simulink library "dspadpt2"  (Simulink 3.00)
libraries: simulink3 x5, dspbdsp2 x5, dspmtrx2 x5, dspbuff2 x3, dspvect2 x1
settings Model: Creator=don  LastModifiedBy=sconahan

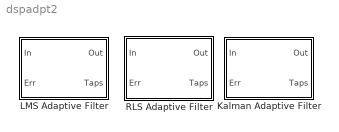
== system dspadpt2 ==
  Kalman Adaptive Filter : Subsystem  mask(Kalman Adaptive Filter){Ntaps=5, Jmin=0.3, q=0.1, ic0=0, K0=0.5, Adapt=off}
      mask prompts: Ntaps "FIR filter length:"; Jmin "Measurement noise variance:"; q "Process noise variance:"; ic0 "Initial value of filter taps:"; K0 "Initial error correlation matrix:"; Adapt "Adapt input"
      mask help: One-step Kalman predictor algorithm for adaptive FIR filtering of input signal. If Adapt input checkbox is enabled, and the Adapt input port is zero, the algorithm stops adapting the filter coefficients.
      mask init:
      | if prod(size(ic0))==1, ic = ic0(ones(Ntaps,1)); else ic = ic0; end
      | if prod(size(K0))==1, K = K0.*eye(Ntaps);
      | elseif any(size(K0)==1), K = diag(K0);
      | else K=K0; end
      | dspblkadpt('init');
      mask Help: web(dspbhelp);
      mask Display: disp('Kalman')
  LMS Adaptive Filter : Subsystem  mask(LMS Adaptive Filter){n=32, mu=.65, ic=0.0, normalized=on, Adapt=off}
      mask prompts: n "FIR filter length:"; mu "Step-size, mu:"; ic "Initial value of filter taps:"; normalized "Use normalization"; Adapt "Adapt input"
      mask help: Least mean-square (LMS) algorithm for adaptive FIR filtering of input signal. Energy normalization may optionally be disabled. If Adapt input checkbox is enabled, and the Adapt input port is zero, the algorithm stops adapting the filter coefficients.
      mask init:
      | if normalized, s='nLMS'; else s='LMS'; end
      | dspblkadpt('init');
      mask Help: web(dspbhelp);
      mask Display: disp(s);
  RLS Adaptive Filter : Subsystem  mask(RLS Adaptive Filter){Ntaps=32, Lambda=1.0, ic=0.0, phi0=0.1, Adapt=off}
      mask prompts: Ntaps "FIR filter length:"; Lambda "Memory weighting factor (0 to 1):"; ic "Initial value of filter taps:"; phi0 "Initial input variance estimate:"; Adapt "Adapt input"
      mask help: Exponentially weighted recursive least-squares (RLS) algorithm for adaptive FIR filtering of input signal. If Adapt input checkbox is enabled, and the Adapt input port is zero, the algorithm stops adapting the filter coefficients.
      mask init:
      | dspblkadpt('init');
      mask Help: web(dspbhelp);
      mask Display: disp('RLS')

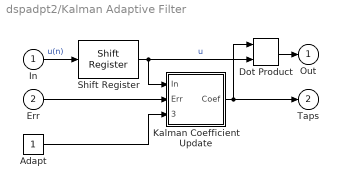
== system dspadpt2/Kalman Adaptive Filter ==
  In : Inport  Port=1  PortWidth=-1  SampleTime=-1  DataType=auto
      settings: SignalType=auto
  Err : Inport  Port=2  PortWidth=-1  SampleTime=-1  DataType=auto
      settings: SignalType=auto
  Adapt : Constant  Value=1
  Dot Product : simulink3/Math/Dot Product
  Kalman Coefficient Update : Subsystem
  Shift Register : dspbuff2/Shift Register  siz=Ntaps  ic=0
  Out : Outport  Port=1  InitialOutput=0
  Taps : Outport  Port=2  InitialOutput=0
  wires:
  In/1 -> Shift Register/1  "u(n)"
  Dot Product/1 -> Out/1
  Err/1 -> Kalman Coefficient Update/2(Err)
  Adapt/1 -> Kalman Coefficient Update/3(Adapt)
  Shift Register/1 -> Kalman Coefficient Update/1(In), Dot Product/2  "u"
  Kalman Coefficient Update/1(Coef) -> Taps/1, Dot Product/1

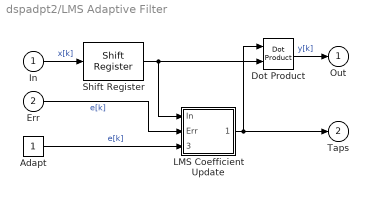
== system dspadpt2/LMS Adaptive Filter ==
  In : Inport  Port=1  PortWidth=-1  SampleTime=-1  DataType=auto
      settings: SignalType=auto
  Err : Inport  Port=2  PortWidth=-1  SampleTime=-1  DataType=auto
      settings: SignalType=auto
  Adapt : Constant  Value=1
  Dot Product : simulink3/Math/Dot Product
  LMS Coefficient Update : Subsystem
  Shift Register : dspbuff2/Shift Register  siz=n  ic=0
  Out : Outport  Port=1  InitialOutput=0
  Taps : Outport  Port=2  InitialOutput=0
  wires:
  Dot Product/1 -> Out/1  "y[k]"
  In/1 -> Shift Register/1  "x[k]"
  Err/1 -> LMS Coefficient Update/2(Err)  "e[k]"
  Adapt/1 -> LMS Coefficient Update/3(Adapt)  "e[k]"
  LMS Coefficient Update/1(Coef) -> Taps/1, Dot Product/1
  Shift Register/1 -> LMS Coefficient Update/1(In), Dot Product/2

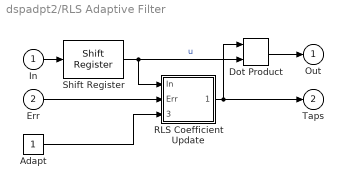
== system dspadpt2/RLS Adaptive Filter ==
  In : Inport  Port=1  PortWidth=-1  SampleTime=-1  DataType=auto
      settings: SignalType=auto
  Err : Inport  Port=2  PortWidth=-1  SampleTime=-1  DataType=auto
      settings: SignalType=auto
  Adapt : Constant  Value=1
  Dot Product : simulink3/Math/Dot Product
  RLS Coefficient Update : Subsystem
  Shift Register : dspbuff2/Shift Register  siz=Ntaps  ic=0
  Out : Outport  Port=1  InitialOutput=0
  Taps : Outport  Port=2  InitialOutput=0
  wires:
  In/1 -> Shift Register/1
  Dot Product/1 -> Out/1
  Err/1 -> RLS Coefficient Update/2(Err)
  Adapt/1 -> RLS Coefficient Update/3(Adapt)
  RLS Coefficient Update/1(Coef) -> Taps/1, Dot Product/1
  Shift Register/1 -> RLS Coefficient Update/1(In), Dot Product/2  "u"

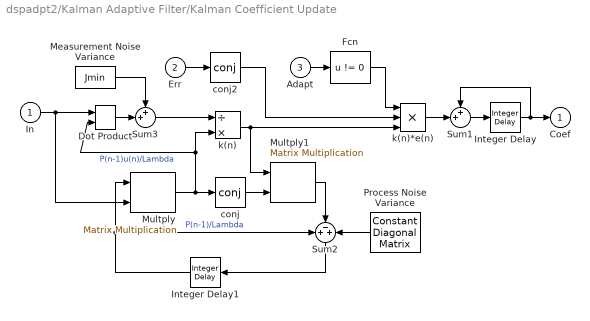
== system dspadpt2/Kalman Adaptive Filter/Kalman Coefficient Update ==
  In : Inport  Port=1  PortWidth=-1  SampleTime=-1  DataType=auto
      settings: SignalType=auto
  Err : Inport  Port=2  PortWidth=-1  SampleTime=-1  DataType=auto
      settings: SignalType=auto
  Adapt : Inport  Port=3  PortWidth=-1  SampleTime=-1  DataType=auto
      settings: SignalType=auto
  Dot Product : simulink3/Math/Dot Product
  Fcn : Fcn  Expr=u != 0
  Integer Delay : dspbdsp2/Integer Delay  delay=1  ic=ic  frame=off  df=on  numChans=1
  Integer Delay1 : dspbdsp2/Integer Delay  Orientation=left  delay=1  ic=K  frame=off  df=on  numChans=1
  Measurement Noise Variance : Constant  Value=Jmin
  Multply : dspmtrx2/Matrix Multiplication  Asize=[Ntaps Ntaps]  Bcols=1
  Multply1 : dspmtrx2/Matrix Multiplication  Asize=[Ntaps 1]  Bcols=Ntaps
  Process Noise Variance : dspmtrx2/Constant Diagonal Matrix  Orientation=left  n=Ntaps  q=q
  Sum1 : Sum  Inputs=++|  SaturateOnIntegerOverflow=on
  Sum2 : Sum  Orientation=down  Inputs=+-+  SaturateOnIntegerOverflow=on
  Sum3 : Sum  Inputs=++|  SaturateOnIntegerOverflow=on
  conj : Math  Operator=conj  OutputSignalType=auto
  conj2 : Math  Operator=conj  OutputSignalType=auto
  k(n) : Product  Inputs=/*  SaturateOnIntegerOverflow=on
  k(n)*e(n) : Product  Inputs=3  SaturateOnIntegerOverflow=on
  Coef : Outport  Port=1  InitialOutput=0
  wires:
  In/1 -> Dot Product/1, Multply/2
  Process Noise Variance/1 -> Sum2/3
  Sum2/1 -> Integer Delay1/1
  Integer Delay1/1 -> Multply/1, Sum2/1  "P(n-1)/Lambda"
  Measurement Noise Variance/1 -> Sum3/1
  Dot Product/1 -> Sum3/2
  Multply1/1 -> Sum2/2
  conj/1 -> Multply1/2
  Multply/1 -> conj/1, k(n)/2, Dot Product/2  "P(n-1)u(n)/Lambda"
  Sum3/1 -> k(n)/1
  k(n)/1 -> Multply1/1, k(n)*e(n)/3
  Err/1 -> conj2/1
  conj2/1 -> k(n)*e(n)/2
  Integer Delay/1 -> Sum1/1, Coef/1
  Sum1/1 -> Integer Delay/1
  k(n)*e(n)/1 -> Sum1/2
  Fcn/1 -> k(n)*e(n)/1
  Adapt/1 -> Fcn/1

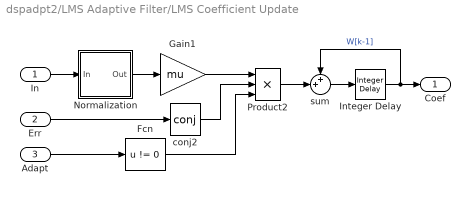
== system dspadpt2/LMS Adaptive Filter/LMS Coefficient Update ==
  In : Inport  Port=1  PortWidth=-1  SampleTime=-1  DataType=auto
      settings: SignalType=auto
  Err : Inport  Port=2  PortWidth=-1  SampleTime=-1  DataType=auto
      settings: SignalType=auto
  Adapt : Inport  Port=3  PortWidth=-1  SampleTime=-1  DataType=auto
      settings: SignalType=auto
  Fcn : Fcn  Expr=u != 0
  Gain1 : Gain  Gain=mu  SaturateOnIntegerOverflow=on
  Integer Delay : dspbdsp2/Integer Delay  delay=1  ic=ic  frame=off  df=on  numChans=1
  Normalization : Subsystem  mask(Replaceable Contents){oname=Normalization, osrc=dspvect2/Normalization, oargs={'NormType','Squared 2-norm','Bias','1e-10'}, replace=~normalized}
      mask prompts: oname "Relative name of blocks to replace:"; osrc "Simulink path to each source block:"; oargs "Parameter/value pairs to each block:"; replace "Replace with short-circuit:"
      mask help: Configurable subsystem holding blocks which may be replaced by virtual short-circuits (muxes) when not needed.
      mask init:
      | opts.name = oname; opts.src = osrc; opts.args = oargs;
      | dspskipblk(gcb,opts,replace);
  Product2 : Product  Inputs=3  SaturateOnIntegerOverflow=on
  conj2 : Math  Operator=conj  OutputSignalType=auto
  sum : Sum  Inputs=++|  SaturateOnIntegerOverflow=on
  Coef : Outport  Port=1  InitialOutput=0
  wires:
  sum/1 -> Integer Delay/1
  conj2/1 -> Product2/2
  Err/1 -> conj2/1
  Gain1/1 -> Product2/1
  Normalization/1(Out) -> Gain1/1
  In/1 -> Normalization/1(In)
  Integer Delay/1 -> Coef/1, sum/1  "W[k-1]"
  Product2/1 -> sum/2
  Adapt/1 -> Fcn/1
  Fcn/1 -> Product2/3

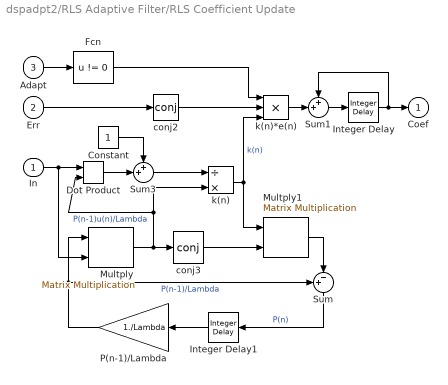
== system dspadpt2/RLS Adaptive Filter/RLS Coefficient Update ==
  In : Inport  Port=1  PortWidth=-1  SampleTime=-1  DataType=auto
      settings: SignalType=auto
  Err : Inport  Port=2  PortWidth=-1  SampleTime=-1  DataType=auto
      settings: SignalType=auto
  Adapt : Inport  Port=3  PortWidth=-1  SampleTime=-1  DataType=auto
      settings: SignalType=auto
  Constant : Constant  Value=1
  Dot Product : simulink3/Math/Dot Product
  Fcn : Fcn  Expr=u != 0
  Integer Delay : dspbdsp2/Integer Delay  delay=1  ic=ic  frame=off  df=on  numChans=1
  Integer Delay1 : dspbdsp2/Integer Delay  Orientation=left  delay=1  ic=eye(Ntaps)./phi0  frame=off  df=on  numChans=1
  Multply : dspmtrx2/Matrix Multiplication  Asize=[Ntaps Ntaps]  Bcols=1
  Multply1 : dspmtrx2/Matrix Multiplication  Asize=[Ntaps 1]  Bcols=Ntaps
  P(n-1)/Lambda : Gain  Orientation=left  Gain=1./Lambda  SaturateOnIntegerOverflow=on
  Sum : Sum  Orientation=down  Inputs=+-|  SaturateOnIntegerOverflow=on
  Sum1 : Sum  Inputs=++|  SaturateOnIntegerOverflow=on
  Sum3 : Sum  Inputs=++|  SaturateOnIntegerOverflow=on
  conj2 : Math  Operator=conj  OutputSignalType=auto
  conj3 : Math  Operator=conj  OutputSignalType=auto
  k(n) : Product  Inputs=/*  SaturateOnIntegerOverflow=on
  k(n)*e(n) : Product  Inputs=3  SaturateOnIntegerOverflow=on
  Coef : Outport  Port=1  InitialOutput=0
  wires:
  Constant/1 -> Sum3/1
  Dot Product/1 -> Sum3/2
  In/1 -> Multply/2, Dot Product/1
  Sum3/1 -> k(n)/1
  Multply/1 -> conj3/1, Dot Product/2, k(n)/2  "P(n-1)u(n)/Lambda"
  conj3/1 -> Multply1/2
  Multply1/1 -> Sum/2
  Integer Delay1/1 -> P(n-1)/Lambda/1
  P(n-1)/Lambda/1 -> Sum/1, Multply/1  "P(n-1)/Lambda"
  Sum/1 -> Integer Delay1/1  "P(n)"
  k(n)/1 -> Multply1/1, k(n)*e(n)/3  "k(n)"
  Err/1 -> conj2/1
  Adapt/1 -> Fcn/1
  conj2/1 -> k(n)*e(n)/2
  Fcn/1 -> k(n)*e(n)/1
  Integer Delay/1 -> Coef/1, Sum1/1
  Sum1/1 -> Integer Delay/1
  k(n)*e(n)/1 -> Sum1/2

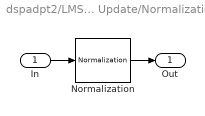
== system dspadpt2/LMS Adaptive Filter/LMS Coefficient Update/Normalization ==
  In : Inport  Port=1  PortWidth=-1  SampleTime=-1  DataType=auto
      settings: SignalType=auto
  Normalization : dspvect2/Normalization  NormType=Squared 2-norm  Bias=1e-10
  Out : Outport  Port=1  InitialOutput=0
  wires:
  In/1 -> Normalization/1
  Normalization/1 -> Out/1
